simulink library "inp"  (Simulink 7.4)
settings: Solver=ode45  StartTime=0.0  StopTime=10.0  RelTol=1e-3
undefined symbols (not defined in the file): AINP_BrkPedalInterp_X_bar, C_TASK_10MS_S, ENUM_SHIFTER_D, ENUM_SHIFTER_N, ENUM_SHIFTER_P, ENUM_SHIFTER_R, KINP_BonnetCloseVehSpdThre_kph, KINP_EDUCoolantTempFilTm_s, KINP_EDUOilPressureFilTm_s, KINP_EDUOilTempFilTm_s, KINP_EDUSynchDisp_mm, KINP_EDUSynchPosnPWMDC_pct_LowerLimit, KINP_EDUSynchPosnPWMDC_pct_ovrdflg, KINP_EDUSynchPosnPWMDC_pct_ovrdval, KINP_EDUSynchPosnPWMDC_pct_UpperLimit, KINP_ShifterPosConfirmD_s, KINP_ShifterPosConfirmN_s, KINP_ShifterPosConfirmP_s, KINP_ShifterPosConfirmR_s, KINP_SingleAccPedalFltRateLim_pct, KINP_TMSpd2VehSpdSigNeg_rpm, KINP_TMSpd2VehSpdSigPos_rpm, KINP_ValidCheck_EDUSynchPosnPWMDC_dec, KINP_ValidCheck_EDUSynchPosnPWMDC_inc, KINP_ValidCheck_EDUSynchPosnPWMDC_lim, KINP_VehSpdSigKeepThres_kph, KPH2MPS, MIN2SEC, MINP_BrkPedalInterp_pct, MPS2KPH, PI, seat_version_control_block_callbacks, TIRE_RADIUS
libraries: inp_lib x166, hcu_lib x4, simulink x1
(part 6 of 9)

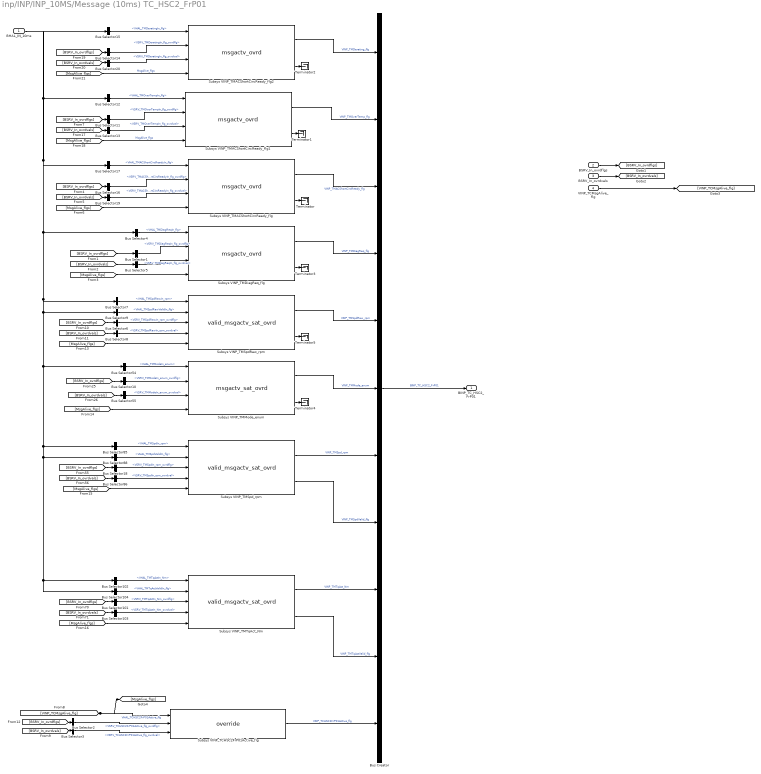
== system inp/INP/INP_10MS/Message (10ms) TC_HSC2_FrP01 ==
  BHAL_IN_10ms : Inport
  BSRV_In_ovrdflgs : Inport  Port=2
  BSRV_In_ovrdvals : Inport  Port=3
  VINP_TCMsgAlive_flg : Inport  Port=4
  Bus Creator : BusCreator  Inputs=11
  Bus Selector1 : BusSelector  OutputSignals=VSRV_TMDiagReqIn_flg_ovrdflg
  Bus Selector10 : BusSelector  OutputSignals=VSRV_TMModeIn_enum_ovrdflg
  Bus Selector101 : BusSelector  OutputSignals=VSRV_TMTqActIn_Nm_ovrdflg
  Bus Selector102 : BusSelector  OutputSignals=VHAL_TMTqActIn_Nm
  Bus Selector103 : BusSelector  OutputSignals=VSRV_TMTqActIn_Nm_ovrdval
  Bus Selector104 : BusSelector  OutputSignals=VHAL_TMTqActValidIn_flg
  Bus Selector11 : BusSelector  OutputSignals=VSRV_TMOverTempIn_flg_ovrdflg
  Bus Selector12 : BusSelector  OutputSignals=VHAL_TMOverTempIn_flg
  Bus Selector13 : BusSelector  OutputSignals=VSRV_TMOverTempIn_flg_ovrdval
  Bus Selector14 : BusSelector  OutputSignals=VSRV_TMDeratingIn_flg_ovrdflg
  Bus Selector15 : BusSelector  OutputSignals=VHAL_TMDeratingIn_flg
  Bus Selector16 : BusSelector  OutputSignals=VSRV_TMACShortCircReadyIn_flg_ovrdflg
  Bus Selector17 : BusSelector  OutputSignals=VHAL_TMACShortCircReadyIn_flg
  Bus Selector18 : BusSelector  OutputSignals=VSRV_TMSpdIn_rpm_ovrdflg
  Bus Selector19 : BusSelector  OutputSignals=VSRV_TMACShortCircReadyIn_flg_ovrdval
  Bus Selector2 : BusSelector  OutputSignals=VSRV_TCHSC2FrP01Active_flg_ovrdflg
  Bus Selector20 : BusSelector  OutputSignals=VSRV_TMDeratingIn_flg_ovrdval
  Bus Selector3 : BusSelector  OutputSignals=VSRV_TCHSC2FrP01Active_flg_ovrdval
  Bus Selector4 : BusSelector  OutputSignals=VHAL_TMDiagReqIn_flg
  Bus Selector5 : BusSelector  OutputSignals=VSRV_TMDiagReqIn_flg_ovrdval
  Bus Selector54 : BusSelector  OutputSignals=VHAL_TMModeIn_enum
  Bus Selector55 : BusSelector  OutputSignals=VSRV_TMModeIn_enum_ovrdval
  Bus Selector6 : BusSelector  OutputSignals=VSRV_TMSpdRawIn_rpm_ovrdflg
  Bus Selector7 : BusSelector  OutputSignals=VHAL_TMSpdRawIn_rpm
  Bus Selector8 : BusSelector  OutputSignals=VSRV_TMSpdRawIn_rpm_ovrdval
  Bus Selector85 : BusSelector  OutputSignals=VHAL_TMSpdIn_rpm
  Bus Selector86 : BusSelector  OutputSignals=VSRV_TMSpdIn_rpm_ovrdval
  Bus Selector88 : BusSelector  OutputSignals=VHAL_TMSpdValidIn_flg
  Bus Selector9 : BusSelector  OutputSignals=VHAL_TMSpdRawValidIn_flg
  Subsys VINP_TCHSC2FrP01Active_flg : inp_lib/override  SystemSampleTime=-1  cal_ovrdflg=KINP_TCHSC2FrP01Active_ovrdflg  cal_ovrdval=KINP_TCHSC2FrP01Active_flg_ovrdval
  Subsys VINP_TMACShortCircReady_flg : inp_lib/msgactv_ovrd  SystemSampleTime=-1  cal_ovrdflg=KINP_TMACShortCircReady_flg_ovrdflg  cal_ovrdval=KINP_TMACShortCircReady_flg_ovrdval  default=KINP_TMACShortCircReadyDefault_flg
  Subsys VINP_TMACShortCircReady_flg1 : inp_lib/msgactv_ovrd  SystemSampleTime=-1  cal_ovrdflg=KINP_TMOverTemp_flg_ovrdflg  cal_ovrdval=KINP_TMOverTemp_flg_ovrdval  default=KINP_TMOverTempDefault_flg
  Subsys VINP_TMACShortCircReady_flg2 : inp_lib/msgactv_ovrd  SystemSampleTime=-1  cal_ovrdflg=KINP_TMDerating_flg_ovrdflg  cal_ovrdval=KINP_TMDerating_flg_ovrdval  default=KINP_TMDeratingDefault_flg
  Subsys VINP_TMDiagReq_flg : inp_lib/msgactv_ovrd  SystemSampleTime=-1  cal_ovrdflg=KINP_TMDiagReq_flg_ovrdflg  cal_ovrdval=KINP_TMDiagReq_flg_ovrdval  default=KINP_TMDiagReqDefault_flg
  Subsys VINP_TMMode_enum : inp_lib/msgactv_sat_ovrd  SystemSampleTime=-1  cal_ovrdflg=KINP_TMMode_enum_ovrdflg  cal_ovrdval=KINP_TMMode_enum_ovrdval  default=KINP_TMModeDefault_enum  hi=KINP_TMMode_enum_Max  lo=KINP_TMMode_enum_Min
  Subsys VINP_TMSpdRaw_rpm : inp_lib/valid_msgactv_sat_ovrd  SystemSampleTime=-1  cal_ovrdflg=KINP_TMSpdRaw_rpm_ovrdflg  cal_ovrdval=KINP_TMSpdRaw_rpm_ovrdval  lim=KINP_ValidCheck_TMSpdRaw_lim  inc=KINP_ValidCheck_TMSpdRaw_inc  dec=KINP_ValidCheck_TMSpdRaw_dec  default=KINP_TMSpdRawDefault_rpm  hi=KINP_TMSpd_rpm_Max  lo=KINP_TMSpd_rpm_Min
  Subsys VINP_TMSpd_rpm : inp_lib/valid_msgactv_sat_ovrd  SystemSampleTime=-1  cal_ovrdflg=KINP_TMSpd_rpm_ovrdflg  cal_ovrdval=KINP_TMSpd_rpm_ovrdval  lim=KINP_ValidCheck_TMSpd_lim  inc=KINP_ValidCheck_TMSpd_inc  dec=KINP_ValidCheck_TMSpd_dec  default=KINP_TMSpdDefault_rpm  hi=KINP_TMSpd_rpm_Max  lo=KINP_TMSpd_rpm_Min
  Subsys VINP_TMTqAct_Nm : inp_lib/valid_msgactv_sat_ovrd  SystemSampleTime=-1  cal_ovrdflg=KINP_TMTqAct_Nm_ovrdflg  cal_ovrdval=KINP_TMTqAct_Nm_ovrdval  lim=KINP_ValidCheck_TMTqAct_lim  inc=KINP_ValidCheck_TMTqAct_inc  dec=KINP_ValidCheck_TMTqAct_dec  default=KINP_TMTqActDefault_Nm  hi=KINP_TMTqAct_Nm_Max  lo=KINP_TMTqAct_Nm_Min
  Terminator{,1..5} (6 alike) : Terminator
  BINP_TC_HSC2_FrP01 : Outport
  wires:
  Bus Creator/1 -> BINP_TC_HSC2_FrP01/1  "BINP_TC_HSC2_FrP01"
  BSRV_In_ovrdvals/1 -> [BSRV_In_ovrdvals]
  BSRV_In_ovrdflgs/1 -> [BSRV_In_ovrdflgs]
  VINP_TCMsgAlive_flg/1 -> [VINP_TCMsgAlive_flg]
  [BSRV_In_ovrdflgs] -> Bus Selector16/1
  [BSRV_In_ovrdvals] -> Bus Selector19/1
  BHAL_IN_10ms/1 -> Bus Selector17/1, Bus Selector7/1, Bus Selector9/1, Bus Selector54/1, Bus Selector85/1, Bus Selector88/1, Bus Selector102/1, Bus Selector104/1, Bus Selector4/1, Bus Selector12/1, Bus Selector15/1
  [VINP_TCMsgAlive_flg] -> [MsgAlive_flgs], Subsys VINP_TCHSC2FrP01Active_flg/1  "VHAL_TCHSC2FrP01Active_flg"
  [BSRV_In_ovrdflgs] -> Bus Selector2/1
  [BSRV_In_ovrdvals] -> Bus Selector3/1
  [BSRV_In_ovrdflgs] -> Bus Selector1/1
  [BSRV_In_ovrdvals] -> Bus Selector5/1
  [BSRV_In_ovrdvals] -> Bus Selector8/1
  [BSRV_In_ovrdflgs] -> Bus Selector6/1
  [BSRV_In_ovrdvals] -> Bus Selector103/1
  [BSRV_In_ovrdflgs] -> Bus Selector101/1
  [BSRV_In_ovrdvals] -> Bus Selector86/1
  [BSRV_In_ovrdflgs] -> Bus Selector18/1
  [BSRV_In_ovrdvals] -> Bus Selector55/1
  [BSRV_In_ovrdflgs] -> Bus Selector10/1
  [BSRV_In_ovrdflgs] -> Bus Selector11/1
  [BSRV_In_ovrdvals] -> Bus Selector13/1
  [BSRV_In_ovrdflgs] -> Bus Selector14/1
  [BSRV_In_ovrdvals] -> Bus Selector20/1
  Bus Selector2/1 -> Subsys VINP_TCHSC2FrP01Active_flg/2  "<VSRV_TCHSC2FrP01Active_flg_ovrdflg>"
  Bus Selector3/1 -> Subsys VINP_TCHSC2FrP01Active_flg/3  "<VSRV_TCHSC2FrP01Active_flg_ovrdval>"
  Subsys VINP_TCHSC2FrP01Active_flg/1 -> Bus Creator/11  "VINP_TCHSC2FrP01Active_flg"
  Bus Selector17/1 -> Subsys VINP_TMACShortCircReady_flg/1  "<VHAL_TMACShortCircReadyIn_flg>"
  Bus Selector16/1 -> Subsys VINP_TMACShortCircReady_flg/2  "<VSRV_TMACShortCircReadyIn_flg_ovrdflg>"
  Bus Selector19/1 -> Subsys VINP_TMACShortCircReady_flg/3  "<VSRV_TMACShortCircReadyIn_flg_ovrdval>"
  [MsgAlive_flgs] -> Subsys VINP_TMACShortCircReady_flg/4
  Subsys VINP_TMACShortCircReady_flg/1 -> Bus Creator/3  "VINP_TMACShortCircReady_flg"
  Subsys VINP_TMACShortCircReady_flg/2 -> Terminator/1
  Bus Selector12/1 -> Subsys VINP_TMACShortCircReady_flg1/1  "<VHAL_TMOverTempIn_flg>"
  Bus Selector11/1 -> Subsys VINP_TMACShortCircReady_flg1/2  "<VSRV_TMOverTempIn_flg_ovrdflg>"
  Bus Selector13/1 -> Subsys VINP_TMACShortCircReady_flg1/3  "<VSRV_TMOverTempIn_flg_ovrdval>"
  [MsgAlive_flgs] -> Subsys VINP_TMACShortCircReady_flg1/4  "MsgAlive_flgs"
  Subsys VINP_TMACShortCircReady_flg1/1 -> Bus Creator/2  "VINP_TMOverTemp_flg"
  Subsys VINP_TMACShortCircReady_flg1/2 -> Terminator1/1
  Bus Selector15/1 -> Subsys VINP_TMACShortCircReady_flg2/1  "<VHAL_TMDeratingIn_flg>"
  Bus Selector14/1 -> Subsys VINP_TMACShortCircReady_flg2/2  "<VSRV_TMDeratingIn_flg_ovrdflg>"
  Bus Selector20/1 -> Subsys VINP_TMACShortCircReady_flg2/3  "<VSRV_TMDeratingIn_flg_ovrdval>"
  [MsgAlive_flgs] -> Subsys VINP_TMACShortCircReady_flg2/4  "MsgAlive_flgs"
  Subsys VINP_TMACShortCircReady_flg2/1 -> Bus Creator/1  "VINP_TMDerating_flg"
  Subsys VINP_TMACShortCircReady_flg2/2 -> Terminator2/1
  Bus Selector4/1 -> Subsys VINP_TMDiagReq_flg/1  "<VHAL_TMDiagReqIn_flg>"
  Bus Selector1/1 -> Subsys VINP_TMDiagReq_flg/2  "<VSRV_TMDiagReqIn_flg_ovrdflg>"
  Bus Selector5/1 -> Subsys VINP_TMDiagReq_flg/3  "<VSRV_TMDiagReqIn_flg_ovrdval>"
  [MsgAlive_flgs] -> Subsys VINP_TMDiagReq_flg/4
  Subsys VINP_TMDiagReq_flg/1 -> Bus Creator/4  "VINP_TMDiagReq_flg"
  Subsys VINP_TMDiagReq_flg/2 -> Terminator3/1
  Bus Selector54/1 -> Subsys VINP_TMMode_enum/1  "<VHAL_TMModeIn_enum>"
  Bus Selector10/1 -> Subsys VINP_TMMode_enum/2  "<VSRV_TMModeIn_enum_ovrdflg>"
  Bus Selector55/1 -> Subsys VINP_TMMode_enum/3  "<VSRV_TMModeIn_enum_ovrdval>"
  [MsgAlive_flgs] -> Subsys VINP_TMMode_enum/4
  Subsys VINP_TMMode_enum/1 -> Bus Creator/6  "VINP_TMMode_enum"
  Subsys VINP_TMMode_enum/2 -> Terminator4/1
  Bus Selector7/1 -> Subsys VINP_TMSpdRaw_rpm/1  "<VHAL_TMSpdRawIn_rpm>"
  Bus Selector9/1 -> Subsys VINP_TMSpdRaw_rpm/2  "<VHAL_TMSpdRawValidIn_flg>"
  Bus Selector6/1 -> Subsys VINP_TMSpdRaw_rpm/3  "<VSRV_TMSpdRawIn_rpm_ovrdflg>"
  Bus Selector8/1 -> Subsys VINP_TMSpdRaw_rpm/4  "<VSRV_TMSpdRawIn_rpm_ovrdval>"
  [MsgAlive_flgs] -> Subsys VINP_TMSpdRaw_rpm/5
  Subsys VINP_TMSpdRaw_rpm/1 -> Bus Creator/5  "VINP_TMSpdRaw_rpm"
  Subsys VINP_TMSpdRaw_rpm/2 -> Terminator5/1
  Bus Selector85/1 -> Subsys VINP_TMSpd_rpm/1  "<VHAL_TMSpdIn_rpm>"
  Bus Selector88/1 -> Subsys VINP_TMSpd_rpm/2  "<VHAL_TMSpdValidIn_flg>"
  Bus Selector18/1 -> Subsys VINP_TMSpd_rpm/3  "<VSRV_TMSpdIn_rpm_ovrdflg>"
  Bus Selector86/1 -> Subsys VINP_TMSpd_rpm/4  "<VSRV_TMSpdIn_rpm_ovrdval>"
  [MsgAlive_flgs] -> Subsys VINP_TMSpd_rpm/5
  Subsys VINP_TMSpd_rpm/1 -> Bus Creator/7  "VINP_TMSpd_rpm"
  Subsys VINP_TMSpd_rpm/2 -> Bus Creator/8  "VINP_TMSpdValid_flg"
  Bus Selector102/1 -> Subsys VINP_TMTqAct_Nm/1  "<VHAL_TMTqActIn_Nm>"
  Bus Selector104/1 -> Subsys VINP_TMTqAct_Nm/2  "<VHAL_TMTqActValidIn_flg>"
  Bus Selector101/1 -> Subsys VINP_TMTqAct_Nm/3  "<VSRV_TMTqActIn_Nm_ovrdflg>"
  Bus Selector103/1 -> Subsys VINP_TMTqAct_Nm/4  "<VSRV_TMTqActIn_Nm_ovrdval>"
  [MsgAlive_flgs] -> Subsys VINP_TMTqAct_Nm/5
  Subsys VINP_TMTqAct_Nm/1 -> Bus Creator/9  "VINP_TMTqAct_Nm"
  Subsys VINP_TMTqAct_Nm/2 -> Bus Creator/10  "VINP_TMTqActValid_flg"

== system inp/INP/INP_10MS/Message (10ms) TC_HSC2_FrP02 ==
  BHAL_IN_10ms : Inport
  BSRV_In_ovrdflgs : Inport  Port=2
  BSRV_In_ovrdvals : Inport  Port=3
  VINP_TCMsgAlive_flg : Inport  Port=4
  Bus Creator : BusCreator
  Bus Selector1 : BusSelector  OutputSignals=VHAL_TMTqAvailMinValidIn_flg
  Bus Selector10 : BusSelector  OutputSignals=VSRV_TMInvtCurrIn_A_ovrdflg
  Bus Selector105 : BusSelector  OutputSignals=VHAL_TMTqAvailMinIn_Nm
  Bus Selector106 : BusSelector  OutputSignals=VSRV_TMTqAvailMinIn_Nm_ovrdval
  Bus Selector109 : BusSelector  OutputSignals=VSRV_TMTqAvailMaxIn_Nm_ovrdval
  Bus Selector112 : BusSelector  OutputSignals=VSRV_TMTqAvailMaxIn_Nm_ovrdflg
  Bus Selector2 : BusSelector  OutputSignals=VSRV_TCHSC2FrP02Active_flg_ovrdflg
  Bus Selector24 : BusSelector  OutputSignals=VSRV_TMTqAvailMinIn_Nm_ovrdflg
  Bus Selector25 : BusSelector  OutputSignals=VHAL_TMTqAvailMaxIn_Nm
  Bus Selector3 : BusSelector  OutputSignals=VSRV_TCHSC2FrP02Active_flg_ovrdval
  Bus Selector4 : BusSelector  OutputSignals=VHAL_TMInvtCurrValidIn_flg
  Bus Selector5 : BusSelector  OutputSignals=VHAL_TMTqAvailMaxValidIn_flg
  Bus Selector8 : BusSelector  OutputSignals=VHAL_TMInvtCurrIn_A
  Bus Selector9 : BusSelector  OutputSignals=VSRV_TMInvtCurrIn_A_ovrdval
  Subsys VINP_TCHSC2FrP02Active_flg : inp_lib/override  SystemSampleTime=-1  cal_ovrdflg=KINP_TCHSC2FrP02Active_ovrdflg  cal_ovrdval=KINP_TCHSC2FrP02Active_flg_ovrdval
  Subsys VINP_TMTqAvailMax_Nm : inp_lib/valid_msgactv_sat_ovrd  SystemSampleTime=-1  cal_ovrdflg=KINP_TMTqAvailMax_Nm_ovrdflg  cal_ovrdval=KINP_TMTqAvailMax_Nm_ovrdval  lim=KINP_ValidCheck_TMTqAvailMax_lim  inc=KINP_ValidCheck_TMTqAvailMax_inc  dec=KINP_ValidCheck_TMTqAvailMax_dec  default=KINP_TMTqAvailMaxDefault_Nm  hi=KINP_TMTqAvailMax_Nm_Max  lo=KINP_TMTqAvailMax_Nm_Min
  Subsys VINP_TMTqAvailMin_Nm : inp_lib/valid_msgactv_sat_ovrd  SystemSampleTime=-1  cal_ovrdflg=KINP_TMTqAvailMin_Nm_ovrdflg  cal_ovrdval=KINP_TMTqAvailMin_Nm_ovrdval  lim=KINP_ValidCheck_TMTqAvailMin_lim  inc=KINP_ValidCheck_TMTqAvailMin_inc  dec=KINP_ValidCheck_TMTqAvailMin_dec  default=KINP_TMTqAvailMinDefault_Nm  hi=KINP_TMTqAvailMin_Nm_Max  lo=KINP_TMTqAvailMin_Nm_Min
  Subsys VINP_VINP_TMInvtCurr_A : inp_lib/valid_msgactv_sat_ovrd  SystemSampleTime=-1  cal_ovrdflg=KINP_TMInvtCurr_A_ovrdflg  cal_ovrdval=KINP_TMInvtCurr_A_ovrdval  lim=KINP_ValidCheck_TMInvtCurr_lim  inc=KINP_ValidCheck_TMInvtCurr_inc  dec=KINP_ValidCheck_TMInvtCurr_dec  default=KINP_TMInvtCurrDefault_A  hi=KINP_TMInvtCurr_A_Max  lo=KINP_TMInvtCurr_A_Min
  Terminator : Terminator
  Terminator1 : Terminator
  Terminator2 : Terminator
  BINP_TC_HSC2_FrP02 : Outport
  wires:
  Bus Selector4/1 -> Subsys VINP_VINP_TMInvtCurr_A/2  "<VHAL_TMInvtCurrValidIn_flg>"
  Bus Selector10/1 -> Subsys VINP_VINP_TMInvtCurr_A/3  "<VSRV_TMInvtCurrIn_A_ovrdflg>"
  BSRV_In_ovrdvals/1 -> [BSRV_In_ovrdvals]
  BSRV_In_ovrdflgs/1 -> [BSRV_In_ovrdflgs]
  VINP_TCMsgAlive_flg/1 -> [VINP_TCMsgAlive_flg]
  Bus Creator/1 -> BINP_TC_HSC2_FrP02/1  "BINP_TC_HSC2_FrP02"
  BHAL_IN_10ms/1 -> Bus Selector105/1, Bus Selector1/1, Bus Selector25/1, Bus Selector4/1, Bus Selector8/1, Bus Selector5/1
  [BSRV_In_ovrdflgs] -> Bus Selector24/1
  [BSRV_In_ovrdvals] -> Bus Selector106/1
  [BSRV_In_ovrdflgs] -> Bus Selector112/1
  [BSRV_In_ovrdvals] -> Bus Selector109/1
  [BSRV_In_ovrdflgs] -> Bus Selector2/1
  [BSRV_In_ovrdvals] -> Bus Selector3/1
  [BSRV_In_ovrdflgs] -> Bus Selector10/1
  [BSRV_In_ovrdvals] -> Bus Selector9/1
  Bus Selector2/1 -> Subsys VINP_TCHSC2FrP02Active_flg/2  "<VSRV_TCHSC2FrP02Active_flg_ovrdflg>"
  Bus Selector3/1 -> Subsys VINP_TCHSC2FrP02Active_flg/3  "<VSRV_TCHSC2FrP02Active_flg_ovrdval>"
  Subsys VINP_TCHSC2FrP02Active_flg/1 -> Bus Creator/4  "VINP_TCHSC2FrP02Active_flg"
  Bus Selector8/1 -> Subsys VINP_VINP_TMInvtCurr_A/1  "<VHAL_TMInvtCurrIn_A>"
  Bus Selector9/1 -> Subsys VINP_VINP_TMInvtCurr_A/4  "<VSRV_TMInvtCurrIn_A_ovrdval>"
  [MsgAlive_flgs] -> Subsys VINP_VINP_TMInvtCurr_A/5
  Subsys VINP_VINP_TMInvtCurr_A/1 -> Bus Creator/3  "VINP_TMInvtCurr_A"
  Subsys VINP_VINP_TMInvtCurr_A/2 -> Terminator/1
  Bus Selector25/1 -> Subsys VINP_TMTqAvailMax_Nm/1  "<VHAL_TMTqAvailMaxIn_Nm>"
  Bus Selector5/1 -> Subsys VINP_TMTqAvailMax_Nm/2  "<VHAL_TMTqAvailMaxValidIn_flg>"
  Bus Selector112/1 -> Subsys VINP_TMTqAvailMax_Nm/3  "<VSRV_TMTqAvailMaxIn_Nm_ovrdflg>"
  Bus Selector109/1 -> Subsys VINP_TMTqAvailMax_Nm/4  "<VSRV_TMTqAvailMaxIn_Nm_ovrdval>"
  [MsgAlive_flgs] -> Subsys VINP_TMTqAvailMax_Nm/5
  Subsys VINP_TMTqAvailMax_Nm/1 -> Bus Creator/2  "VINP_TMTqAvailMax_Nm"
  Subsys VINP_TMTqAvailMax_Nm/2 -> Terminator1/1
  Bus Selector105/1 -> Subsys VINP_TMTqAvailMin_Nm/1  "<VHAL_TMTqAvailMinIn_Nm>"
  Bus Selector1/1 -> Subsys VINP_TMTqAvailMin_Nm/2  "<VHAL_TMTqAvailMinValidIn_flg>"
  Bus Selector24/1 -> Subsys VINP_TMTqAvailMin_Nm/3  "<VSRV_TMTqAvailMinIn_Nm_ovrdflg>"
  Bus Selector106/1 -> Subsys VINP_TMTqAvailMin_Nm/4  "<VSRV_TMTqAvailMinIn_Nm_ovrdval>"
  [MsgAlive_flgs] -> Subsys VINP_TMTqAvailMin_Nm/5
  Subsys VINP_TMTqAvailMin_Nm/1 -> Bus Creator/1  "VINP_TMTqAvailMin_Nm"
  Subsys VINP_TMTqAvailMin_Nm/2 -> Terminator2/1
  [VINP_TCMsgAlive_flg] -> Subsys VINP_TCHSC2FrP02Active_flg/1, [MsgAlive_flgs]  "VINP_TCMsgAlive_flg"

== system inp/INP/INP_10MS/Message (10ms)DSC_HSC_FrP00 ==
  BHAL_IN_10ms : Inport
  BSRV_In_ovrdflgs : Inport  Port=2
  BSRV_In_ovrdvals : Inport  Port=3
  VINP_DSCMsgAlive_flg : Inport  Port=4
  Bus Creator : BusCreator  Inputs=5
  Bus Selector1 : BusSelector  OutputSignals=VHAL_GearShiftInhDownValidIn_flg
  Bus Selector10 : BusSelector  OutputSignals=VHAL_GearShiftInhUpValidIn_flg
  Bus Selector2 : BusSelector  OutputSignals=VSRV_DSCHSCFrP00Active_flg_ovrdflg
  Bus Selector3 : BusSelector  OutputSignals=VHAL_GearShiftInhDownIn_flg
  Bus Selector4 : BusSelector  OutputSignals=VSRV_DSCHSCFrP00Active_flg_ovrdval
  Bus Selector5 : BusSelector  OutputSignals=VSRV_GearShiftInhDownIn_flg_ovrdflg
  Bus Selector6 : BusSelector  OutputSignals=VSRV_GearShiftInhDownIn_flg_ovrdval
  Bus Selector7 : BusSelector  OutputSignals=VHAL_GearShiftInhUpIn_flg
  Bus Selector8 : BusSelector  OutputSignals=VSRV_GearShiftInhUpIn_flg_ovrdflg
  Bus Selector9 : BusSelector  OutputSignals=VSRV_GearShiftInhUpIn_flg_ovrdval
  Subsys VINP_DSCHSCFrP00Active_flg : inp_lib/override  SystemSampleTime=-1  cal_ovrdflg=KINP_DSCHSCFrP00Active_ovrdflg  cal_ovrdval=KINP_DSCHSCFrP00Active_flg_ovrdval
  Subsys VINP_GearShiftInhDown_flg : inp_lib/valid_msgactv_ovrd  SystemSampleTime=-1  cal_ovrdflg=KINP_GearShiftInhDown_flg_ovrdflg  cal_ovrdval=KINP_GearShiftInhDown_flg_ovrdval  lim=KINP_ValidCheck_GearShiftInhDown_lim  inc=KINP_ValidCheck_GearShiftInhDown_inc  dec=KINP_ValidCheck_GearShiftInhDown_dec  default=KINP_GearShiftInhDownDefault_flg
  Subsys VINP_GearShiftInhUp_flg : inp_lib/valid_msgactv_ovrd  SystemSampleTime=-1  cal_ovrdflg=KINP_GearShiftInhUp_flg_ovrdflg  cal_ovrdval=KINP_GearShiftInhUp_flg_ovrdval  lim=KINP_ValidCheck_GearShiftInhUp_lim  inc=KINP_ValidCheck_GearShiftInhUp_inc  dec=KINP_ValidCheck_GearShiftInhUp_dec  default=KINP_GearShiftInhUpDefault_flg
  BINP_DSC_HSC_FrP00 : Outport  OutDataType=sfix(16)  OutScaling=2^0
  wires:
  [MsgAlive_flgs] -> Subsys VINP_GearShiftInhUp_flg/5
  Bus Selector9/1 -> Subsys VINP_GearShiftInhUp_flg/4  "<VSRV_GearShiftInhUpIn_flg_ovrdval>"
  Bus Selector8/1 -> Subsys VINP_GearShiftInhUp_flg/3  "<VSRV_GearShiftInhUpIn_flg_ovrdflg>"
  Bus Selector10/1 -> Subsys VINP_GearShiftInhUp_flg/2  "<VHAL_GearShiftInhUpValidIn_flg>"
  Bus Selector5/1 -> Subsys VINP_GearShiftInhDown_flg/3  "<VSRV_GearShiftInhDownIn_flg_ovrdflg>"
  Bus Selector1/1 -> Subsys VINP_GearShiftInhDown_flg/2  "<VHAL_GearShiftInhDownValidIn_flg>"
  [BSRV_In_ovrdflgs] -> Bus Selector8/1
  [BSRV_In_ovrdvals] -> Bus Selector9/1
  BHAL_IN_10ms/1 -> Bus Selector1/1, Bus Selector10/1, Bus Selector7/1, Bus Selector3/1
  [BSRV_In_ovrdflgs] -> Bus Selector5/1
  [BSRV_In_ovrdvals] -> Bus Selector6/1
  Bus Creator/1 -> BINP_DSC_HSC_FrP00/1  "BINP_DSC_HSC_FrP00"
  BSRV_In_ovrdvals/1 -> [BSRV_In_ovrdvals]
  BSRV_In_ovrdflgs/1 -> [BSRV_In_ovrdflgs]
  VINP_DSCMsgAlive_flg/1 -> [VINP_DSCMsgAlive_flg]
  [VINP_DSCMsgAlive_flg] -> [MsgAlive_flgs], Subsys VINP_DSCHSCFrP00Active_flg/1  "VHAL_DSCHSCFrP00Active_flg"
  [BSRV_In_ovrdflgs] -> Bus Selector2/1
  [BSRV_In_ovrdvals] -> Bus Selector4/1
  Bus Selector2/1 -> Subsys VINP_DSCHSCFrP00Active_flg/2  "<VSRV_DSCHSCFrP00Active_flg_ovrdflg>"
  Bus Selector4/1 -> Subsys VINP_DSCHSCFrP00Active_flg/3  "<VSRV_DSCHSCFrP00Active_flg_ovrdval>"
  Subsys VINP_DSCHSCFrP00Active_flg/1 -> Bus Creator/5  "VINP_DSCHSCFrP00Active_flg"
  Bus Selector3/1 -> Subsys VINP_GearShiftInhDown_flg/1  "<VHAL_GearShiftInhDownIn_flg>"
  Bus Selector6/1 -> Subsys VINP_GearShiftInhDown_flg/4  "<VSRV_GearShiftInhDownIn_flg_ovrdval>"
  [MsgAlive_flgs] -> Subsys VINP_GearShiftInhDown_flg/5
  Subsys VINP_GearShiftInhDown_flg/1 -> Bus Creator/1  "VINP_GearShiftInhDown_flg"
  Subsys VINP_GearShiftInhDown_flg/2 -> Bus Creator/2  "VINP_GearShiftInhDownValid_flg"
  Bus Selector7/1 -> Subsys VINP_GearShiftInhUp_flg/1  "<VHAL_GearShiftInhUpIn_flg>"
  Subsys VINP_GearShiftInhUp_flg/1 -> Bus Creator/3  "VINP_GearShiftInhUp_flg"
  Subsys VINP_GearShiftInhUp_flg/2 -> Bus Creator/4  "VINP_GearShiftInhUpValid_flg"

== system inp/INP/INP_10MS/Message (10ms)DSC_HSC_FrP02 ==
  BHAL_IN_10ms : Inport
  BSRV_In_ovrdflgs : Inport  Port=2
  BSRV_In_ovrdvals : Inport  Port=3
  VINP_DSCMsgAlive_flg : Inport  Port=4
  Bus Selector1 : BusSelector  OutputSignals=VHAL_ESPTqIncControlActiveIn_flg
  Bus Selector2 : BusSelector  OutputSignals=VSRV_DSCHSCFrP02Active_flg_ovrdflg
  Bus Selector20 : BusSelector  OutputSignals=VSRV_ESPTqIncControlActiveIn_flg_ovrdflg
  Bus Selector23 : BusSelector  OutputSignals=VSRV_ESPTqIncControlActiveIn_flg_ovrdval
  Bus Selector3 : BusSelector  OutputSignals=VSRV_DSCHSCFrP02Active_flg_ovrdval
  Bus Selector33 : BusSelector  OutputSignals=VHAL_ESPTqRedControlActiveIn_flg
  Bus Selector35 : BusSelector  OutputSignals=VSRV_ESPTqRedControlActiveIn_flg_ovrdflg
  Bus Selector36 : BusSelector  OutputSignals=VSRV_ESPTqRedControlActiveIn_flg_ovrdval
  Bus Selector37 : BusSelector  OutputSignals=VSRV_ESPTqIncSlowReqIn_Nm_ovrdval
  Bus Selector38 : BusSelector  OutputSignals=VHAL_ESPTqIncSlowReqIn_Nm
  Bus Selector4 : BusSelector  OutputSignals=VHAL_ESPTqIncSlowReqValidIn_flg
  Bus Selector40 : BusSelector  OutputSignals=VSRV_ESPTqIncSlowReqIn_Nm_ovrdflg
  Bus Selector41 : BusSelector  OutputSignals=VSRV_ESPTqRedFastReqIn_Nm_ovrdval
  Bus Selector42 : BusSelector  OutputSignals=VHAL_ESPTqRedFastReqIn_Nm
  Bus Selector44 : BusSelector  OutputSignals=VSRV_ESPTqRedFastReqIn_Nm_ovrdflg
  Bus Selector45 : BusSelector  OutputSignals=VSRV_ESPTqRedSlowReqIn_Nm_ovrdval
  Bus Selector46 : BusSelector  OutputSignals=VHAL_ESPTqRedSlowReqIn_Nm
  Bus Selector48 : BusSelector  OutputSignals=VSRV_ESPTqRedSlowReqIn_Nm_ovrdflg
  Bus Selector5 : BusSelector  OutputSignals=VHAL_ESPTqRedSlowReqValidIn_flg
  Bus Selector6 : BusSelector  OutputSignals=VHAL_ESPTqRedFastReqValidIn_flg
  Subsys VINP_DSCHSCFrP02Active_flg : inp_lib/override  SystemSampleTime=-1  cal_ovrdflg=KINP_DSCHSCFrP02Active_ovrdflg  cal_ovrdval=KINP_DSCHSCFrP02Active_flg_ovrdval
  Subsys VINP_ESPTqIncControlActive_flg : inp_lib/msgactv_ovrd  SystemSampleTime=-1  cal_ovrdflg=KINP_ESPTqIncControlActive_flg_ovrdflg  cal_ovrdval=KINP_ESPTqIncControlActive_flg_ovrdval  default=KINP_ESPTqIncControlActiveDefault_flg
  Subsys VINP_ESPTqIncSlowReq_Nm : inp_lib/valid_msgactv_sat_ovrd  SystemSampleTime=-1  cal_ovrdflg=KINP_ESPTqIncSlowReq_Nm_ovrdflg  cal_ovrdval=KINP_ESPTqIncSlowReq_Nm_ovrdval  lim=KINP_ValidCheck_ESPTqIncSlowReq_lim  inc=KINP_ValidCheck_ESPTqIncSlowReq_inc  dec=KINP_ValidCheck_ESPTqIncSlowReq_dec  default=KINP_ESPTqIncSlowReqDefault_Nm  hi=KINP_ESPTqIncSlowReq_Nm_Max  lo=KINP_ESPTqIncSlowReq_Nm_Min
  Subsys VINP_ESPTqRedFastReq_Nm : inp_lib/valid_msgactv_sat_ovrd  SystemSampleTime=-1  cal_ovrdflg=KINP_ESPTqRedFastReq_Nm_ovrdflg  cal_ovrdval=KINP_ESPTqRedFastReq_Nm_ovrdval  lim=KINP_ValidCheck_ESPTqRedFastReq_lim  inc=KINP_ValidCheck_ESPTqRedFastReq_inc  dec=KINP_ValidCheck_ESPTqRedFastReq_dec  default=KINP_ESPTqRedFastReqDefault_Nm  hi=KINP_ESPTqRedFastReq_Nm_Max  lo=KINP_ESPTqRedFastReq_Nm_Min
  Subsys VINP_ESPTqRedReqActive_flg : inp_lib/msgactv_ovrd  SystemSampleTime=-1  cal_ovrdflg=KINP_ESPTqRedControlActive_flg_ovrdflg  cal_ovrdval=KINP_ESPTqRedControlActive_flg_ovrdval  default=KINP_ESPTqRedControlActiveDefault_flg
  Subsys VINP_ESPTqRedSlowReq_Nm : inp_lib/valid_msgactv_sat_ovrd  SystemSampleTime=-1  cal_ovrdflg=KINP_ESPTqRedSlowReq_Nm_ovrdflg  cal_ovrdval=KINP_ESPTqRedSlowReq_Nm_ovrdval  lim=KINP_ValidCheck_ESPTqRedSlowReq_lim  inc=KINP_ValidCheck_ESPTqRedSlowReq_inc  dec=KINP_ValidCheck_ESPTqRedSlowReq_dec  default=KINP_ESPTqRedSlowReqDefault_Nm  hi=KINP_ESPTqRedSlowReq_Nm_Max  lo=KINP_ESPTqRedSlowReq_Nm_Min
  Terminator{,1..4} (5 alike) : Terminator
  inputs_bus1 : BusCreator  Inputs=6
  BINP_DSC_HSC_FrP02 : Outport  OutDataType=sfix(16)  OutScaling=2^0
  wires:
  Bus Selector6/1 -> Subsys VINP_ESPTqRedFastReq_Nm/2  "<VHAL_ESPTqRedFastReqValidIn_flg>"
  Bus Selector5/1 -> Subsys VINP_ESPTqRedSlowReq_Nm/2  "<VHAL_ESPTqRedSlowReqValidIn_flg>"
  Bus Selector48/1 -> Subsys VINP_ESPTqRedSlowReq_Nm/3  "<VSRV_ESPTqRedSlowReqIn_Nm_ovrdflg>"
  Bus Selector44/1 -> Subsys VINP_ESPTqRedFastReq_Nm/3  "<VSRV_ESPTqRedFastReqIn_Nm_ovrdflg>"
  Bus Selector4/1 -> Subsys VINP_ESPTqIncSlowReq_Nm/2  "<VHAL_ESPTqIncSlowReqValidIn_flg>"
  [BSRV_In_ovrdvals] -> Bus Selector23/1
  [BSRV_In_ovrdflgs] -> Bus Selector20/1
  [BSRV_In_ovrdvals] -> Bus Selector36/1
  [BSRV_In_ovrdflgs] -> Bus Selector35/1
  [BSRV_In_ovrdvals] -> Bus Selector37/1
  [BSRV_In_ovrdvals] -> Bus Selector41/1
  [BSRV_In_ovrdflgs] -> Bus Selector44/1
  [BSRV_In_ovrdvals] -> Bus Selector45/1
  [BSRV_In_ovrdflgs] -> Bus Selector48/1
  VINP_DSCMsgAlive_flg/1 -> [VINP_DSCMsgAlive_flg]
  BSRV_In_ovrdflgs/1 -> [BSRV_In_ovrdflgs]
  BSRV_In_ovrdvals/1 -> [BSRV_In_ovrdvals]
  inputs_bus1/1 -> BINP_DSC_HSC_FrP02/1  "BINP_DSC_HSC_FrP02"
  BHAL_IN_10ms/1 -> Bus Selector1/1, Bus Selector4/1, Bus Selector6/1, Bus Selector5/1, Bus Selector46/1, Bus Selector42/1, Bus Selector38/1, Bus Selector33/1
  [BSRV_In_ovrdflgs] -> Bus Selector40/1
  [VINP_DSCMsgAlive_flg] -> [MsgAlive_flgs], Subsys VINP_DSCHSCFrP02Active_flg/1
  [BSRV_In_ovrdflgs] -> Bus Selector2/1
  [BSRV_In_ovrdvals] -> Bus Selector3/1
  Bus Selector2/1 -> Subsys VINP_DSCHSCFrP02Active_flg/2  "<VSRV_DSCHSCFrP02Active_flg_ovrdflg>"
  Bus Selector3/1 -> Subsys VINP_DSCHSCFrP02Active_flg/3  "<VSRV_DSCHSCFrP02Active_flg_ovrdval>"
  Subsys VINP_DSCHSCFrP02Active_flg/1 -> inputs_bus1/6  "VINP_DSCHSCFrP02Active_flg"
  Bus Selector1/1 -> Subsys VINP_ESPTqIncControlActive_flg/1  "<VHAL_ESPTqIncControlActiveIn_flg>"
  Bus Selector20/1 -> Subsys VINP_ESPTqIncControlActive_flg/2  "<VSRV_ESPTqIncControlActiveIn_flg_ovrdflg>"
  Bus Selector23/1 -> Subsys VINP_ESPTqIncControlActive_flg/3  "<VSRV_ESPTqIncControlActiveIn_flg_ovrdval>"
  [MsgAlive_flgs] -> Subsys VINP_ESPTqIncControlActive_flg/4
  Subsys VINP_ESPTqIncControlActive_flg/1 -> inputs_bus1/1  "VINP_ESPTqIncControlActive_flg"
  Subsys VINP_ESPTqIncControlActive_flg/2 -> Terminator/1
  Bus Selector38/1 -> Subsys VINP_ESPTqIncSlowReq_Nm/1  "<VHAL_ESPTqIncSlowReqIn_Nm>"
  Bus Selector40/1 -> Subsys VINP_ESPTqIncSlowReq_Nm/3  "<VSRV_ESPTqIncSlowReqIn_Nm_ovrdflg>"
  Bus Selector37/1 -> Subsys VINP_ESPTqIncSlowReq_Nm/4  "<VSRV_ESPTqIncSlowReqIn_Nm_ovrdval>"
  [MsgAlive_flgs] -> Subsys VINP_ESPTqIncSlowReq_Nm/5
  Subsys VINP_ESPTqIncSlowReq_Nm/1 -> inputs_bus1/3  "VINP_ESPTqIncSlowReq_Nm"
  Subsys VINP_ESPTqIncSlowReq_Nm/2 -> Terminator1/1
  Bus Selector42/1 -> Subsys VINP_ESPTqRedFastReq_Nm/1  "<VHAL_ESPTqRedFastReqIn_Nm>"
  Bus Selector41/1 -> Subsys VINP_ESPTqRedFastReq_Nm/4  "<VSRV_ESPTqRedFastReqIn_Nm_ovrdval>"
  [MsgAlive_flgs] -> Subsys VINP_ESPTqRedFastReq_Nm/5
  Subsys VINP_ESPTqRedFastReq_Nm/1 -> inputs_bus1/4  "VINP_ESPTqRedFastReq_Nm"
  Subsys VINP_ESPTqRedFastReq_Nm/2 -> Terminator2/1
  Bus Selector33/1 -> Subsys VINP_ESPTqRedReqActive_flg/1  "<VHAL_ESPTqRedControlActiveIn_flg>"
  Bus Selector35/1 -> Subsys VINP_ESPTqRedReqActive_flg/2  "<VSRV_ESPTqRedControlActiveIn_flg_ovrdflg>"
  Bus Selector36/1 -> Subsys VINP_ESPTqRedReqActive_flg/3  "<VSRV_ESPTqRedControlActiveIn_flg_ovrdval>"
  [MsgAlive_flgs] -> Subsys VINP_ESPTqRedReqActive_flg/4
  Subsys VINP_ESPTqRedReqActive_flg/1 -> inputs_bus1/2  "VINP_ESPTqRedControlActive_flg"
  Subsys VINP_ESPTqRedReqActive_flg/2 -> Terminator3/1
  Bus Selector46/1 -> Subsys VINP_ESPTqRedSlowReq_Nm/1  "<VHAL_ESPTqRedSlowReqIn_Nm>"
  Bus Selector45/1 -> Subsys VINP_ESPTqRedSlowReq_Nm/4  "<VSRV_ESPTqRedSlowReqIn_Nm_ovrdval>"
  [MsgAlive_flgs] -> Subsys VINP_ESPTqRedSlowReq_Nm/5
  Subsys VINP_ESPTqRedSlowReq_Nm/1 -> inputs_bus1/5  "VINP_ESPTqRedSlowReq_Nm"
  Subsys VINP_ESPTqRedSlowReq_Nm/2 -> Terminator4/1

== system inp/INP/INP_20MS/BSRV_In_ovrdflgs ==
  Constant: VSRV_AccPedSingleFltIn_flg_ovrdflg : Constant  Value=0  OutDataTypeMode=boolean  OutDataTypeStr=boolean
  Constant: VSRV_BMSChrgBufferValidIn_flg_ovrdflg : Constant  Value=0  OutDataTypeMode=boolean  OutDataTypeStr=boolean
  Constant: VSRV_BMSDchaBufferIn_pct_ovrdflg : Constant  Value=0  OutDataTypeMode=boolean  OutDataTypeStr=boolean
  Constant: VSRV_BMSDchaBufferValidIn_flg_ovrdflg : Constant  Value=0  OutDataTypeMode=boolean  OutDataTypeStr=boolean
  Constant: VSRV_BMSHSC2FrP03Active_flg_ovrdflg : Constant  Value=0  OutDataTypeMode=boolean  OutDataTypeStr=boolean
  Constant: VSRV_BMSHSC2FrP03ProtFault_flg_ovrdflg : Constant  Value=0  OutDataTypeMode=boolean  OutDataTypeStr=boolean
  Constant: VSRV_BMSPeakChrgPwrIn_kW_ovrdflg : Constant  Value=0  OutDataTypeMode=boolean  OutDataTypeStr=boolean
  Constant: VSRV_BMSPeakChrgPwrValidIn_flg_ovrdflg : Constant  Value=0  OutDataTypeMode=boolean  OutDataTypeStr=boolean
  Constant: VSRV_BMSPeakDchaPwrIn_kW_ovrdflg : Constant  Value=0  OutDataTypeMode=boolean  OutDataTypeStr=boolean
  Constant: VSRV_BMSPeakDchaPwrValidIn_flg_ovrdflg : Constant  Value=0  OutDataTypeMode=boolean  OutDataTypeStr=boolean
  Constant: VSRV_BrkVacPumpStateIn_enum_ovrdflg : Constant  Value=0  OutDataTypeMode=boolean  OutDataTypeStr=boolean
  Constant: VSRV_CruiseControlActiveIn_flg_ovrdflg : Constant  Value=0  OutDataTypeMode=boolean  OutDataTypeStr=boolean
  Constant: VSRV_DSCHSCFrP04Active_flg_ovrdflg : Constant  Value=0  OutDataTypeMode=boolean  OutDataTypeStr=boolean
  Constant: VSRV_EDUOilPressureIn_bar_ovrdflg : Constant  Value=0  OutDataTypeMode=boolean  OutDataTypeStr=boolean
  Constant: VSRV_EDUOilPressureValidIn_flg_ovrdflg : Constant  Value=0  OutDataTypeMode=boolean  OutDataTypeStr=boolean
  Constant: VSRV_EMSHSCFrP01Active_flg_ovrdflg : Constant  Value=0  OutDataTypeMode=boolean  OutDataTypeStr=boolean
  Constant: VSRV_EMSHSCFrP03Active_flg_ovrdflg : Constant  Value=0  OutDataTypeMode=boolean  OutDataTypeStr=boolean
  Constant: VSRV_EPBHSCFrP00Active_flg_ovrdflg : Constant  Value=0  OutDataTypeMode=boolean  OutDataTypeStr=boolean
  Constant: VSRV_EPBHSCFrP00ProtFault_flg_ovrdflg : Constant  Value=0  OutDataTypeMode=boolean  OutDataTypeStr=boolean
  Constant: VSRV_EPBStatusIn_enum_ovrdflg : Constant  Value=0  OutDataTypeMode=boolean  OutDataTypeStr=boolean
  Constant: VSRV_ESPRegenFaultIn_flg_ovrdflg : Constant  Value=0  OutDataTypeMode=boolean  OutDataTypeStr=boolean
  Constant: VSRV_ESPRegenTargetIn_Nm_ovrdflg : Constant  Value=0  OutDataTypeMode=boolean  OutDataTypeStr=boolean
  Constant: VSRV_ESPRegenTargetValidIn_flg_ovrdflg : Constant  Value=0  OutDataTypeMode=boolean  OutDataTypeStr=boolean
  Constant: VSRV_EngAutoStopInhibitIn_flg_ovrdflg : Constant  Value=0  OutDataTypeMode=boolean  OutDataTypeStr=boolean
  Constant: VSRV_EngCoolantTempIn_C_ovrdflg : Constant  Value=0  OutDataTypeMode=boolean  OutDataTypeStr=boolean
  Constant: VSRV_EngCoolantTempValidIn_flg_ovrdflg : Constant  Value=0  OutDataTypeMode=boolean  OutDataTypeStr=boolean
  Constant: VSRV_EngIdleTypeReqIn_enum_ovrdflg : Constant  Value=0  OutDataTypeMode=boolean  OutDataTypeStr=boolean
  Constant: VSRV_FuelConsumptionCurrentValue_ovrdflg : Constant  Value=0  OutDataTypeMode=boolean  OutDataTypeStr=boolean
  Constant: VSRV_GSensorIn_g_ovrdflg : Constant  Value=0  OutDataTypeMode=boolean  OutDataTypeStr=boolean
  Constant: VSRV_HVBattBalanceReqIn_flg_ovrdflg : Constant  Value=0  OutDataTypeMode=boolean  OutDataTypeStr=boolean
  Constant: VSRV_HVBattChargeCurrMaxIn_A_ovrdflg : Constant  Value=0  OutDataTypeMode=boolean  OutDataTypeStr=boolean
  Constant: VSRV_HVBattChargeCurrMaxValidIn_flg_ovrdflg : Constant  Value=0  OutDataTypeMode=boolean  OutDataTypeStr=boolean
  Constant: VSRV_HVBattDischargeCurrMaxIn_A_ovrdflg : Constant  Value=0  OutDataTypeMode=boolean  OutDataTypeStr=boolean
  Constant: VSRV_HVBattDischargeCurrMaxValidIn_flg_ovrdflg : Constant  Value=0  OutDataTypeMode=boolean  OutDataTypeStr=boolean
  Constant: VSRV_HVBattEnergyAvailIn_kWh_ovrdflg : Constant  Value=0  OutDataTypeMode=boolean  OutDataTypeStr=boolean
  Constant: VSRV_HVBattPwrAvailChargeIn_kW_ovrdflg : Constant  Value=0  OutDataTypeMode=boolean  OutDataTypeStr=boolean
  Constant: VSRV_HVBattPwrAvailChargeValidIn_flg_ovrdflg : Constant  Value=0  OutDataTypeMode=boolean  OutDataTypeStr=boolean
  Constant: VSRV_HVBattPwrAvailDischargeIn_kW_ovrdflg : Constant  Value=0  OutDataTypeMode=boolean  OutDataTypeStr=boolean
  Constant: VSRV_HVBattPwrAvailDischargeValidIn_flg_ovrdflg : Constant  Value=0  OutDataTypeMode=boolean  OutDataTypeStr=boolean
  Constant: VSRV_SMUHSCFrP02Active_flg_ovrdflg : Constant  Value=0  OutDataTypeMode=boolean  OutDataTypeStr=boolean
  Constant: VSRV_SecurityKeyValidIn_flg_ovrdflg : Constant  Value=0  OutDataTypeMode=boolean  OutDataTypeStr=boolean
  Constant:VSRV_ACCPedFltIn_flg_ovrdflg : Constant  Value=0  OutDataTypeMode=boolean  OutDataTypeStr=boolean
  Constant:VSRV_BMSChrgBufferIn_pct_ovrdflg : Constant  Value=0  OutDataTypeMode=boolean  OutDataTypeStr=boolean
  Constant:VSRV_EngStartReqIn_enum_ovrdflg : Constant  Value=0  OutDataTypeMode=boolean  OutDataTypeStr=boolean
  Constant:VSRV_HVBattEnergyAvailValidIn_flg_ovrdflg : Constant  Value=0  OutDataTypeMode=boolean  OutDataTypeStr=boolean
  Constant:VSRV_HVBattFltLampOnReqIn_flg_ovrdflg : Constant  Value=0  OutDataTypeMode=boolean  OutDataTypeStr=boolean
  inputs_bus : BusCreator  Inputs=46
  output_bus : Outport
  wires:
  Constant: VSRV_EDUOilPressureIn_bar_ovrdflg/1 -> inputs_bus/45  "VSRV_EDUOilPressureIn_bar_ovrdflg"
  Constant: VSRV_EDUOilPressureValidIn_flg_ovrdflg/1 -> inputs_bus/46  "VSRV_EDUOilPressureValidIn_flg_ovrdflg"
  Constant: VSRV_BMSDchaBufferValidIn_flg_ovrdflg/1 -> inputs_bus/44  "VSRV_BMSDchaBufferValidIn_flg_ovrdflg"
  Constant: VSRV_BMSDchaBufferIn_pct_ovrdflg/1 -> inputs_bus/43  "VSRV_BMSDchaBufferIn_pct_ovrdflg"
  Constant: VSRV_BMSChrgBufferValidIn_flg_ovrdflg/1 -> inputs_bus/42  "VSRV_BMSChrgBufferValidIn_flg_ovrdflg"
  Constant:VSRV_BMSChrgBufferIn_pct_ovrdflg/1 -> inputs_bus/41  "VSRV_BMSChrgBufferIn_pct_ovrdflg"
  Constant: VSRV_BMSPeakDchaPwrValidIn_flg_ovrdflg/1 -> inputs_bus/40  "VSRV_BMSPeakDchaPwrValidIn_flg_ovrdflg"
  Constant: VSRV_BMSPeakDchaPwrIn_kW_ovrdflg/1 -> inputs_bus/39  "VSRV_BMSPeakDchaPwrIn_kW_ovrdflg"
  Constant: VSRV_BMSPeakChrgPwrValidIn_flg_ovrdflg/1 -> inputs_bus/38  "VSRV_BMSPeakChrgPwrValidIn_flg_ovrdflg"
  Constant: VSRV_BMSPeakChrgPwrIn_kW_ovrdflg/1 -> inputs_bus/37  "VSRV_BMSPeakChrgPwrIn_kW_ovrdflg"
  Constant: VSRV_HVBattPwrAvailDischargeValidIn_flg_ovrdflg/1 -> inputs_bus/36  "VSRV_HVBattPwrAvailDischargeValidIn_flg_ovrdflg"
  Constant: VSRV_HVBattPwrAvailDischargeIn_kW_ovrdflg/1 -> inputs_bus/35  "VSRV_HVBattPwrAvailDischargeIn_kW_ovrdflg"
  Constant: VSRV_HVBattPwrAvailChargeValidIn_flg_ovrdflg/1 -> inputs_bus/34  "VSRV_HVBattPwrAvailChargeValidIn_flg_ovrdflg"
  Constant: VSRV_HVBattPwrAvailChargeIn_kW_ovrdflg/1 -> inputs_bus/33  "VSRV_HVBattPwrAvailChargeIn_kW_ovrdflg"
  Constant:VSRV_ACCPedFltIn_flg_ovrdflg/1 -> inputs_bus/32  "VSRV_ACCPedFltIn_flg_ovrdflg"
  Constant:VSRV_EngStartReqIn_enum_ovrdflg/1 -> inputs_bus/31  "VSRV_EngStartReqIn_enum_ovrdflg"
  Constant:VSRV_HVBattFltLampOnReqIn_flg_ovrdflg/1 -> inputs_bus/30  "VSRV_HVBattFltLampOnReqIn_flg_ovrdflg"
  Constant: VSRV_HVBattBalanceReqIn_flg_ovrdflg/1 -> inputs_bus/29  "VSRV_HVBattBalanceReqIn_flg_ovrdflg"
  Constant:VSRV_HVBattEnergyAvailValidIn_flg_ovrdflg/1 -> inputs_bus/28  "VSRV_HVBattEnergyAvailValidIn_flg_ovrdflg"
  Constant: VSRV_HVBattEnergyAvailIn_kWh_ovrdflg/1 -> inputs_bus/27  "VSRV_HVBattEnergyAvailIn_kWh_ovrdflg"
  Constant: VSRV_AccPedSingleFltIn_flg_ovrdflg/1 -> inputs_bus/26  "VSRV_AccPedSingleFltIn_flg_ovrdflg"
  Constant: VSRV_EngIdleTypeReqIn_enum_ovrdflg/1 -> inputs_bus/25  "VSRV_EngIdleTypeReqIn_enum_ovrdflg"
  Constant: VSRV_BrkVacPumpStateIn_enum_ovrdflg/1 -> inputs_bus/24  "VSRV_BrkVacPumpStateIn_enum_ovrdflg"
  Constant: VSRV_CruiseControlActiveIn_flg_ovrdflg/1 -> inputs_bus/23  "VSRV_CruiseControlActiveIn_flg_ovrdflg"
  Constant: VSRV_EPBStatusIn_enum_ovrdflg/1 -> inputs_bus/22  "VSRV_EPBStatusIn_enum_ovrdflg"
  Constant: VSRV_DSCHSCFrP04Active_flg_ovrdflg/1 -> inputs_bus/21  "VSRV_DSCHSCFrP04Active_flg_ovrdflg"
  Constant: VSRV_ESPRegenTargetIn_Nm_ovrdflg/1 -> inputs_bus/20  "VSRV_ESPRegenTargetIn_Nm_ovrdflg"
  Constant: VSRV_SMUHSCFrP02Active_flg_ovrdflg/1 -> inputs_bus/19  "VSRV_SMUHSCFrP02Active_flg_ovrdflg"
  Constant: VSRV_SecurityKeyValidIn_flg_ovrdflg/1 -> inputs_bus/18  "VSRV_SecurityKeyValidIn_flg_ovrdflg"
  Constant: VSRV_ESPRegenFaultIn_flg_ovrdflg/1 -> inputs_bus/17  "VSRV_ESPRegenFaultIn_flg_ovrdflg"
  Constant: VSRV_HVBattDischargeCurrMaxValidIn_flg_ovrdflg/1 -> inputs_bus/16  "VSRV_HVBattDischargeCurrMaxValidIn_flg_ovrdflg"
  Constant: VSRV_HVBattDischargeCurrMaxIn_A_ovrdflg/1 -> inputs_bus/15  "VSRV_HVBattDischargeCurrMaxIn_A_ovrdflg"
  Constant: VSRV_HVBattChargeCurrMaxValidIn_flg_ovrdflg/1 -> inputs_bus/14  "VSRV_HVBattChargeCurrMaxValidIn_flg_ovrdflg"
  Constant: VSRV_HVBattChargeCurrMaxIn_A_ovrdflg/1 -> inputs_bus/13  "VSRV_HVBattChargeCurrMaxIn_A_ovrdflg"
  Constant: VSRV_GSensorIn_g_ovrdflg/1 -> inputs_bus/12  "VSRV_GSensorIn_g_ovrdflg"
  Constant: VSRV_ESPRegenTargetValidIn_flg_ovrdflg/1 -> inputs_bus/11  "VSRV_ESPRegenTargetValidIn_flg_ovrdflg"
  Constant: VSRV_EPBHSCFrP00Active_flg_ovrdflg/1 -> inputs_bus/10  "VSRV_EPBHSCFrP00Active_flg_ovrdflg"
  Constant: VSRV_EngCoolantTempValidIn_flg_ovrdflg/1 -> inputs_bus/9  "VSRV_EngCoolantTempValidIn_flg_ovrdflg"
  Constant: VSRV_EngCoolantTempIn_C_ovrdflg/1 -> inputs_bus/8  "VSRV_EngCoolantTempIn_C_ovrdflg"
  Constant: VSRV_EngAutoStopInhibitIn_flg_ovrdflg/1 -> inputs_bus/7  "VSRV_EngAutoStopInhibitIn_flg_ovrdflg"
  Constant: VSRV_EMSHSCFrP03Active_flg_ovrdflg/1 -> inputs_bus/6  "VSRV_EMSHSCFrP03Active_flg_ovrdflg"
  Constant: VSRV_EMSHSCFrP01Active_flg_ovrdflg/1 -> inputs_bus/5  "VSRV_EMSHSCFrP01Active_flg_ovrdflg"
  Constant: VSRV_BMSHSC2FrP03Active_flg_ovrdflg/1 -> inputs_bus/4  "VSRV_BMSHSC2FrP03Active_flg_ovrdflg"
  Constant: VSRV_FuelConsumptionCurrentValue_ovrdflg/1 -> inputs_bus/3  "VSRV_FuelConsumptionCurrentValue_ovrdflg"
  Constant: VSRV_EPBHSCFrP00ProtFault_flg_ovrdflg/1 -> inputs_bus/2  "VSRV_EPBHSCFrP00ProtFault_flg_ovrdflg"
  Constant: VSRV_BMSHSC2FrP03ProtFault_flg_ovrdflg/1 -> inputs_bus/1  "VSRV_BMSHSC2FrP03ProtFault_flg_ovrdflg"
  inputs_bus/1 -> output_bus/1  "output_bus"

== system inp/INP/INP_20MS/BSRV_in_ovrdvals ==
  Constant: VSRV_AccPedSingleFltIn_flg_ovrdval : Constant  Value=0  OutDataTypeMode=boolean  OutDataTypeStr=boolean
  Constant: VSRV_BMSChrgBufferValidIn_flg_ovrdval : Constant  Value=0  OutDataTypeMode=boolean  OutDataTypeStr=boolean
  Constant: VSRV_BMSDchaBufferIn_pct_ovrdval : Constant  Value=0.0  OutDataTypeMode=single  OutDataTypeStr=single
  Constant: VSRV_BMSDchaBufferValidIn_flg_ovrdval : Constant  Value=0  OutDataTypeMode=boolean  OutDataTypeStr=boolean
  Constant: VSRV_BMSHSC2FrP03Active_flg_ovrdval : Constant  Value=0  OutDataTypeMode=boolean  OutDataTypeStr=boolean
  Constant: VSRV_BMSHSC2FrP03ProtFault_flg_ovrdval : Constant  Value=0  OutDataTypeMode=boolean  OutDataTypeStr=boolean
  Constant: VSRV_BMSPeakChrgPwrIn_kW_ovrdval : Constant  Value=0.0  OutDataTypeMode=single  OutDataTypeStr=single
  Constant: VSRV_BMSPeakChrgPwrValidIn_flg_ovrdval : Constant  Value=0  OutDataTypeMode=boolean  OutDataTypeStr=boolean
  Constant: VSRV_BMSPeakDchaPwrIn_kW_ovrdval : Constant  Value=0.0  OutDataTypeMode=single  OutDataTypeStr=single
  Constant: VSRV_BMSPeakDchaPwrValidIn_flg_ovrdval : Constant  Value=0  OutDataTypeMode=boolean  OutDataTypeStr=boolean
  Constant: VSRV_CruiseControlActiveIn_flg_ovrdval : Constant  Value=0  OutDataTypeMode=boolean  OutDataTypeStr=boolean
  Constant: VSRV_EDUOilPressureIn_bar_ovrdval : Constant  Value=0.0  OutDataTypeMode=single  OutDataTypeStr=single
  Constant: VSRV_EDUOilPressureValidIn_flg_ovrdval : Constant  Value=0  OutDataTypeMode=boolean  OutDataTypeStr=boolean
  Constant: VSRV_EMSHSCFrP01Active_flg_ovrdval : Constant  Value=0  OutDataTypeMode=boolean  OutDataTypeStr=boolean
  Constant: VSRV_EMSHSCFrP03Active_flg_ovrdval : Constant  Value=0  OutDataTypeMode=boolean  OutDataTypeStr=boolean
  Constant: VSRV_EPBHSCFrP00Active_flg_ovrdval : Constant  Value=0  OutDataTypeMode=boolean  OutDataTypeStr=boolean
  Constant: VSRV_EPBHSCFrP00ProtFault_flg_ovrdval : Constant  Value=0  OutDataTypeMode=boolean  OutDataTypeStr=boolean
  Constant: VSRV_ESPRegenFaultIn_flg_ovrdval : Constant  Value=0  OutDataTypeMode=boolean  OutDataTypeStr=boolean
  Constant: VSRV_ESPRegenTargetValidIn_flg_ovrdval : Constant  Value=0  OutDataTypeMode=boolean  OutDataTypeStr=boolean
  Constant: VSRV_EngAutoStopInhibitIn_flg_ovrdval : Constant  Value=0  OutDataTypeMode=boolean  OutDataTypeStr=boolean
  Constant: VSRV_EngCoolantTempIn_C_ovrdval : Constant  Value=0.0  OutDataTypeMode=single  OutDataTypeStr=single
  Constant: VSRV_EngCoolantTempValidIn_flg_ovrdval : Constant  Value=0  OutDataTypeMode=boolean  OutDataTypeStr=boolean
  Constant: VSRV_EngIdleTypeReqIn_enum_ovrdval : Constant  Value=0  OutDataTypeMode=uint8  OutDataTypeStr=uint8
  Constant: VSRV_FuelConsumptionCurrentValue_ovrdval : Constant  Value=0.0  OutDataTypeMode=single  OutDataTypeStr=single
  Constant: VSRV_GSensorIn_g_ovrdval : Constant  Value=0.0  OutDataTypeMode=single  OutDataTypeStr=single
  Constant: VSRV_HVBattChargeCurrMaxIn_A_ovrdval : Constant  Value=0.0  OutDataTypeMode=single  OutDataTypeStr=single
  Constant: VSRV_HVBattChargeCurrMaxValidIn_flg_ovrdval : Constant  Value=0  OutDataTypeMode=boolean  OutDataTypeStr=boolean
  Constant: VSRV_HVBattDischargeCurrMaxIn_A_ovrdval : Constant  Value=0.0  OutDataTypeMode=single  OutDataTypeStr=single
  Constant: VSRV_HVBattDischargeCurrMaxValidIn_flg_ovrdval : Constant  Value=0  OutDataTypeMode=boolean  OutDataTypeStr=boolean
  Constant: VSRV_HVBattEnergyAvailIn_kWh_ovrdval : Constant  Value=0  OutDataTypeMode=single  OutDataTypeStr=single
  Constant: VSRV_HVBattPwrAvailChargeIn_kW_ovrdval : Constant  Value=0.0  OutDataTypeMode=single  OutDataTypeStr=single
  Constant: VSRV_HVBattPwrAvailChargeValidIn_flg_ovrdval : Constant  Value=0  OutDataTypeMode=boolean  OutDataTypeStr=boolean
  Constant: VSRV_HVBattPwrAvailDischargeIn_kW_ovrdval : Constant  Value=0.0  OutDataTypeMode=single  OutDataTypeStr=single
  Constant: VSRV_HVBattPwrAvailDischargeValidIn_flg_ovrdval : Constant  Value=0  OutDataTypeMode=boolean  OutDataTypeStr=boolean
  Constant: VSRV_SMUHSCFrP02Active_flg_ovrdval : Constant  Value=0  OutDataTypeMode=boolean  OutDataTypeStr=boolean
  Constant: VSRV_SecurityKeyValidIn_flg_ovrdval : Constant  Value=0  OutDataTypeMode=boolean  OutDataTypeStr=boolean
  Constant:VSRV_ACCPedFltIn_flg_ovrdval : Constant  Value=0  OutDataTypeMode=boolean  OutDataTypeStr=boolean
  Constant:VSRV_BMSChrgBufferIn_pct_ovrdval : Constant  Value=0.0  OutDataTypeMode=single  OutDataTypeStr=single
  Constant:VSRV_BrkVacPumpStateIn_enum_ovrdval : Constant  Value=0  OutDataTypeMode=uint8  OutDataTypeStr=uint8
  Constant:VSRV_DSCHSCFrP04Active_flg_ovrdval : Constant  Value=0  OutDataTypeMode=boolean  OutDataTypeStr=boolean
  Constant:VSRV_EPBStatusIn_enum_ovrdval : Constant  Value=0  OutDataTypeMode=uint8  OutDataTypeStr=uint8
  Constant:VSRV_ESPRegenTargetIn_Nm_ovrdval : Constant  Value=0  OutDataTypeMode=single  OutDataTypeStr=single
  Constant:VSRV_EngStartReqIn_enum_ovrdval : Constant  Value=0  OutDataTypeMode=uint8  OutDataTypeStr=uint8
  Constant:VSRV_HVBattBalanceReqIn_flg_ovrdval : Constant  Value=0  OutDataTypeMode=boolean  OutDataTypeStr=boolean
  Constant:VSRV_HVBattEnergyAvailValidIn_flg_ovrdval : Constant  Value=0  OutDataTypeMode=boolean  OutDataTypeStr=boolean
  Constant:VSRV_HVBattFltLampOnReqIn_flg_ovrdval : Constant  Value=0  OutDataTypeMode=boolean  OutDataTypeStr=boolean
  inputs_bus : BusCreator  Inputs=46
  output_bus : Outport
  wires:
  Constant: VSRV_EDUOilPressureValidIn_flg_ovrdval/1 -> inputs_bus/46  "VSRV_EDUOilPressureValidIn_flg_ovrdval"
  Constant: VSRV_EDUOilPressureIn_bar_ovrdval/1 -> inputs_bus/45  "VSRV_EDUOilPressureIn_bar_ovrdval"
  Constant: VSRV_BMSDchaBufferValidIn_flg_ovrdval/1 -> inputs_bus/44  "VSRV_BMSDchaBufferValidIn_flg_ovrdval"
  Constant: VSRV_BMSDchaBufferIn_pct_ovrdval/1 -> inputs_bus/43  "VSRV_BMSDchaBufferIn_pct_ovrdval"
  Constant: VSRV_BMSChrgBufferValidIn_flg_ovrdval/1 -> inputs_bus/42  "VSRV_BMSChrgBufferValidIn_flg_ovrdval"
  Constant:VSRV_BMSChrgBufferIn_pct_ovrdval/1 -> inputs_bus/41  "VSRV_BMSChrgBufferIn_pct_ovrdval"
  Constant: VSRV_BMSPeakDchaPwrValidIn_flg_ovrdval/1 -> inputs_bus/40  "VSRV_BMSPeakDchaPwrValidIn_flg_ovrdval"
  Constant: VSRV_BMSPeakDchaPwrIn_kW_ovrdval/1 -> inputs_bus/39  "VSRV_BMSPeakDchaPwrIn_kW_ovrdval"
  Constant: VSRV_BMSPeakChrgPwrValidIn_flg_ovrdval/1 -> inputs_bus/38  "VSRV_BMSPeakChrgPwrValidIn_flg_ovrdval"
  Constant: VSRV_BMSPeakChrgPwrIn_kW_ovrdval/1 -> inputs_bus/37  "VSRV_BMSPeakChrgPwrIn_kW_ovrdval"
  Constant: VSRV_HVBattPwrAvailDischargeValidIn_flg_ovrdval/1 -> inputs_bus/36  "VSRV_HVBattPwrAvailDischargeValidIn_flg_ovrdval"
  Constant: VSRV_HVBattPwrAvailDischargeIn_kW_ovrdval/1 -> inputs_bus/35  "VSRV_HVBattPwrAvailDischargeIn_kW_ovrdval"
  Constant: VSRV_HVBattPwrAvailChargeValidIn_flg_ovrdval/1 -> inputs_bus/34  "VSRV_HVBattPwrAvailChargeValidIn_flg_ovrdval"
  Constant: VSRV_HVBattPwrAvailChargeIn_kW_ovrdval/1 -> inputs_bus/33  "VSRV_HVBattPwrAvailChargeIn_kW_ovrdval"
  Constant:VSRV_ACCPedFltIn_flg_ovrdval/1 -> inputs_bus/32  "VSRV_ACCPedFltIn_flg_ovrdval"
  Constant:VSRV_EngStartReqIn_enum_ovrdval/1 -> inputs_bus/31  "VSRV_EngStartReqIn_enum_ovrdval"
  Constant:VSRV_HVBattFltLampOnReqIn_flg_ovrdval/1 -> inputs_bus/30  "VSRV_HVBattFltLampOnReqIn_flg_ovrdval"
  Constant:VSRV_HVBattBalanceReqIn_flg_ovrdval/1 -> inputs_bus/29  "VSRV_HVBattBalanceReqIn_flg_ovrdval"
  Constant:VSRV_HVBattEnergyAvailValidIn_flg_ovrdval/1 -> inputs_bus/28  "VSRV_HVBattEnergyAvailValidIn_flg_ovrdval"
  Constant: VSRV_HVBattEnergyAvailIn_kWh_ovrdval/1 -> inputs_bus/27  "VSRV_HVBattEnergyAvailIn_kWh_ovrdval"
  Constant: VSRV_AccPedSingleFltIn_flg_ovrdval/1 -> inputs_bus/26  "VSRV_AccPedSingleFltIn_flg_ovrdval"
  Constant: VSRV_EngIdleTypeReqIn_enum_ovrdval/1 -> inputs_bus/25  "VSRV_EngIdleTypeReqIn_enum_ovrdval"
  Constant:VSRV_BrkVacPumpStateIn_enum_ovrdval/1 -> inputs_bus/24  "VSRV_BrkVacPumpStateIn_enum_ovrdval"
  Constant: VSRV_CruiseControlActiveIn_flg_ovrdval/1 -> inputs_bus/23  "VSRV_CruiseControlActiveIn_flg_ovrdval"
  Constant:VSRV_EPBStatusIn_enum_ovrdval/1 -> inputs_bus/22  "VSRV_EPBStatusIn_enum_ovrdval"
  Constant:VSRV_DSCHSCFrP04Active_flg_ovrdval/1 -> inputs_bus/21  "VSRV_DSCHSCFrP04Active_flg_ovrdval"
  Constant:VSRV_ESPRegenTargetIn_Nm_ovrdval/1 -> inputs_bus/20  "VSRV_ESPRegenTargetIn_Nm_ovrdval"
  Constant: VSRV_SMUHSCFrP02Active_flg_ovrdval/1 -> inputs_bus/19  "VSRV_SMUHSCFrP02Active_flg_ovrdval"
  Constant: VSRV_SecurityKeyValidIn_flg_ovrdval/1 -> inputs_bus/18  "VSRV_SecurityKeyValidIn_flg_ovrdval"
  Constant: VSRV_ESPRegenFaultIn_flg_ovrdval/1 -> inputs_bus/17  "VSRV_ESPRegenFaultIn_flg_ovrdval"
  Constant: VSRV_HVBattDischargeCurrMaxValidIn_flg_ovrdval/1 -> inputs_bus/16  "VSRV_HVBattDischargeCurrMaxValidIn_flg_ovrdval"
  Constant: VSRV_HVBattDischargeCurrMaxIn_A_ovrdval/1 -> inputs_bus/15  "VSRV_HVBattDischargeCurrMaxIn_A_ovrdval"
  Constant: VSRV_HVBattChargeCurrMaxValidIn_flg_ovrdval/1 -> inputs_bus/14  "VSRV_HVBattChargeCurrMaxValidIn_flg_ovrdval"
  Constant: VSRV_HVBattChargeCurrMaxIn_A_ovrdval/1 -> inputs_bus/13  "VSRV_HVBattChargeCurrMaxIn_A_ovrdval"
  Constant: VSRV_GSensorIn_g_ovrdval/1 -> inputs_bus/12  "VSRV_GSensorIn_g_ovrdval"
  Constant: VSRV_ESPRegenTargetValidIn_flg_ovrdval/1 -> inputs_bus/11  "VSRV_ESPRegenTargetValidIn_flg_ovrdval"
  Constant: VSRV_EPBHSCFrP00Active_flg_ovrdval/1 -> inputs_bus/10  "VSRV_EPBHSCFrP00Active_flg_ovrdval"
  Constant: VSRV_EngCoolantTempValidIn_flg_ovrdval/1 -> inputs_bus/9  "VSRV_EngCoolantTempValidIn_flg_ovrdval"
  Constant: VSRV_EngCoolantTempIn_C_ovrdval/1 -> inputs_bus/8  "VSRV_EngCoolantTempIn_C_ovrdval"
  Constant: VSRV_EngAutoStopInhibitIn_flg_ovrdval/1 -> inputs_bus/7  "VSRV_EngAutoStopInhibitIn_flg_ovrdval"
  Constant: VSRV_EMSHSCFrP03Active_flg_ovrdval/1 -> inputs_bus/6  "VSRV_EMSHSCFrP03Active_flg_ovrdval"
  Constant: VSRV_EMSHSCFrP01Active_flg_ovrdval/1 -> inputs_bus/5  "VSRV_EMSHSCFrP01Active_flg_ovrdval"
  Constant: VSRV_BMSHSC2FrP03Active_flg_ovrdval/1 -> inputs_bus/4  "VSRV_BMSHSC2FrP03Active_flg_ovrdval"
  Constant: VSRV_FuelConsumptionCurrentValue_ovrdval/1 -> inputs_bus/3  "VSRV_FuelConsumptionCurrentValue_ovrdval"
  Constant: VSRV_EPBHSCFrP00ProtFault_flg_ovrdval/1 -> inputs_bus/2  "VSRV_EPBHSCFrP00ProtFault_flg_ovrdval"
  Constant: VSRV_BMSHSC2FrP03ProtFault_flg_ovrdval/1 -> inputs_bus/1  "VSRV_BMSHSC2FrP03ProtFault_flg_ovrdval"
  inputs_bus/1 -> output_bus/1  "output_bus_ovrdval"
